simulink model "test_2"  (R2014a)
settings: Solver=ode45  StartTime=0.0  StopTime=20  RelTol=1e-3
libraries: simulink x1
settings Model: Creator=BIgC46263347  LastModifiedBy=BIgC46263347

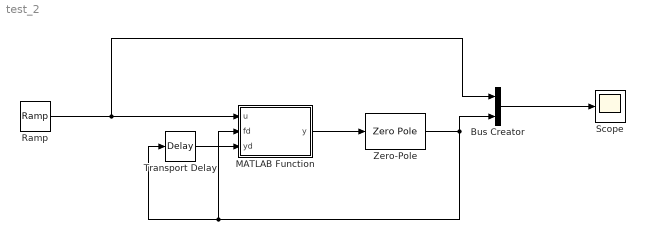
== system test_2 ==
  Bus Creator : BusCreator  Inputs=2
  MATLAB Function : MATLAB Function  TreatAsAtomicUnit=on
  Ramp : simulink/Sources/Ramp  slope=1  start=0  X0=0
  Scope : Scope
  Transport Delay : TransportDelay
  Zero-Pole : ZeroPole  Zeros=[]  Poles=[-1/20]  Gain=[1/10]
  wires:
  Bus Creator/1 -> Scope/1
  MATLAB Function/1(y) -> Zero-Pole/1
  Ramp/1 -> Bus Creator/1, MATLAB Function/1(u)
  Zero-Pole/1 -> Bus Creator/2, Transport Delay/1, MATLAB Function/2(fd)
  Transport Delay/1 -> MATLAB Function/3(yd)

== matlab function test_2/MATLAB Function ==
  data: u input; y output; fd input; yd input
function y = fcn(u,fd,yd)
rf=3;
gap=0.5;


y=yd;
if(fd>(rf+gap))
   y=0;
elseif(fd<(rf+gap))
   y=u;
end


end
